simulink model "DDEF_Nylon_fwr"  (R2026a)
settings: Solver=ode45  StopTime=10  MaxStep=1e-4  RelTol=1e-6
undefined symbols (not defined in the file): RL
libraries: fl_lib x5, ee_lib x4, nesl_utility x4, simulink x1
settings Model: Creator=Satyanarayan  LastModifiedBy=Satyanarayan

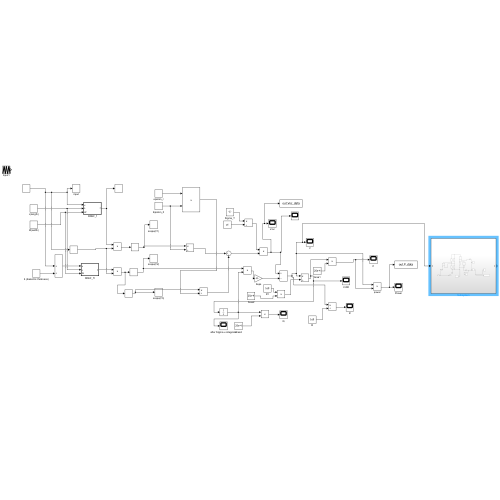
[thumbnail: Simulink's stored preview of the top-level diagram]
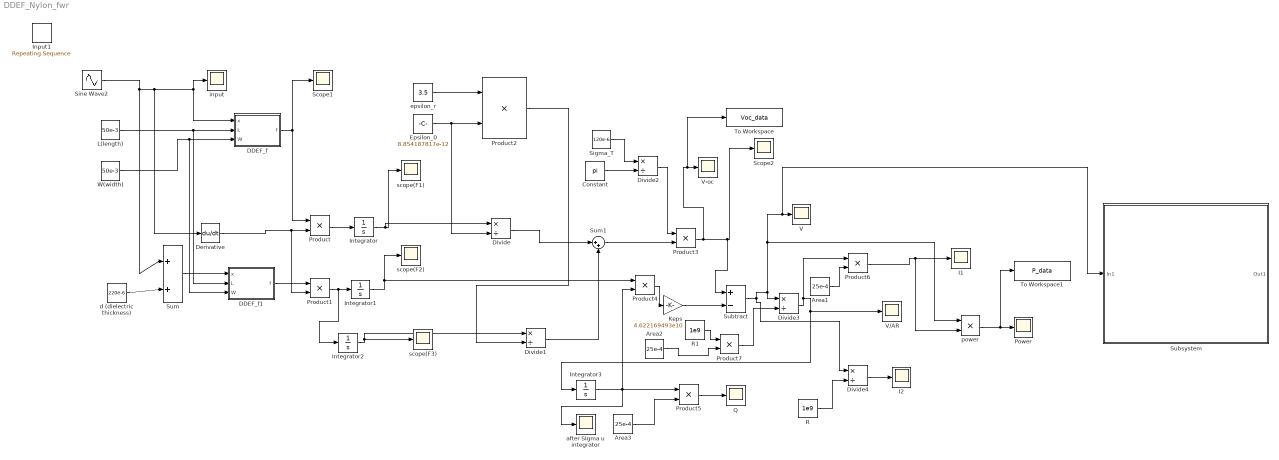
== system DDEF_Nylon_fwr ==
  Area1 : Constant  Value=25e-4
  Area2 : Constant  Value=25e-4
  Area3 : Constant  Value=25e-4
  Constant : Constant  Value=pi
  DDEF_f : MATLAB Function  TreatAsAtomicUnit=on
  DDEF_f1 : MATLAB Function  TreatAsAtomicUnit=on
  Derivative : Derivative
  Divide{,1..4} (5 alike) : Product  Inputs=*/
  Epsilon_0 : Constant  Value=8.854187817e-12
  I1 : Scope
      settings: ActiveDisplayYMinimum=-1  ActiveDisplayYMaximum=1  DataLoggingVariableName=ScopeData11
  I2 : Scope
      settings: ActiveDisplayYMinimum=-1  ActiveDisplayYMaximum=1  DataLoggingVariableName=ScopeData12
  Input1 : simulink/Sources/Repeating Sequence  rep_seq_t=[0 0.5 1]  rep_seq_y=[0 0.01 0]
  Integrator : Integrator
  Integrator1 : Integrator  InitialCondition=3.44206e-4
  Integrator2 : Integrator
  Integrator3 : Integrator
  Keps : Gain  Gain=4.622169493e10
  L(length) : Constant  Value=50e-3
  Power : Scope
      settings: ActiveDisplayYMinimum=-0.00046209975030593484  ActiveDisplayYMaximum=0.0041588977527534142  DataLoggingVariableName=ScopeData13
  Product{,1..7} (8 alike) : Product
  Q : Scope
      settings: ActiveDisplayYMinimum=-1  ActiveDisplayYMaximum=1  DataLoggingVariableName=ScopeData10
  R : Constant  Value=1e9
  R1 : Constant  Value=1e9
  Scope1 : Scope
      settings: ActiveDisplayYMinimum=0.392699081716402  ActiveDisplayYMaximum=1.7016960205353724
  Scope2 : Scope
      settings: ActiveDisplayYMinimum=-1  ActiveDisplayYMaximum=1  DataLoggingVariableName=ScopeData5
  Sigma_T : Constant  Value=120e-6
  Sine Wave2 : Sin  Amplitude=2.5e-3  Bias=2.5e-3  Frequency=2*pi  Phase=3*pi/2  SampleTime=0
  Subsystem : Subsystem
  Subtract : Sum  Inputs=+-
  Sum : Sum  Inputs=|++
  Sum1 : Sum  Inputs=|++
  To Workspace : ToWorkspace  VariableName=Voc_data  SaveFormat=Timeseries  SampleTime=-1
  To Workspace1 : ToWorkspace  VariableName=P_data  SaveFormat=Timeseries  SampleTime=-1
  V : Scope
      settings: ActiveDisplayYMinimum=-1408.9203660031535  ActiveDisplayYMaximum=2630.0910844886675  DataLoggingVariableName=ScopeData6
  V-oc : Scope
      settings: ActiveDisplayYMinimum=-4819.8788285773553  ActiveDisplayYMaximum=43269.459838287345  DataLoggingVariableName=ScopeData9
  V/AR : Scope
      settings: ActiveDisplayYMinimum=-1  ActiveDisplayYMaximum=1  DataLoggingVariableName=ScopeData8
  W(width) : Constant  Value=50e-3
  after SIgma u integrator : Scope
      settings: ActiveDisplayYMinimum=-3.4716855225550229E-6  ActiveDisplayYMaximum=3.1245169702995217E-5  DataLoggingVariableName=ScopeData7
  d (dielectric thickness) : Constant  Value=220e-6
  epsilon_r : Constant  Value=3.5
  input : Scope
      settings: ActiveDisplayYMinimum=-0.0012499995532938208  ActiveDisplayYMaximum=0.011249995979644389
  power : Product
  scope(F1) : Scope
      settings: ActiveDisplayYMinimum=-0.00121173424121706  ActiveDisplayYMaximum=0.01090560817095354  DataLoggingVariableName=ScopeData2
  scope(F2) : Scope
      settings: ActiveDisplayYMinimum=0.00041232627300281824  ActiveDisplayYMaximum=0.01127511879777789  DataLoggingVariableName=ScopeData3
  scope(F3) : Scope
      settings: ActiveDisplayYMinimum=-0.0010878737269972396  ActiveDisplayYMaximum=0.009774918797777957  DataLoggingVariableName=ScopeData4
  wires:
  Area1/1 -> Product6/2
  Divide2/1 -> Product3/1
  Product4/1 -> Keps/1
  Divide4/1 -> I2/1
  Divide/1 -> Sum1/1
  Sigma_T/1 -> Divide2/1
  Keps/1 -> Subtract/2
  Divide3/1 -> Product6/1, Integrator3/1, V/AR/1
  Sum/1 -> DDEF_f1/1(x)
  d (dielectric thickness)/1 -> Sum/2
  Product/1 -> Integrator/1
  Derivative/1 -> Product1/2, Product/2
  Integrator/1 -> Divide/1, scope(F1)/1
  Product3/1 -> To Workspace/1, V-oc/1, Subtract/1, Scope2/1
  Constant/1 -> Divide2/2
  Product7/1 -> Divide3/2
  Integrator2/1 -> Divide1/1, scope(F3)/1
  Product5/1 -> Q/1
  Sine Wave2/1 -> Sum/1, Derivative/1, DDEF_f/1(x), input/1
  R/1 -> Divide4/2
  power/1 -> To Workspace1/1, Power/1
  Area3/1 -> Product5/2
  Integrator3/1 -> Product5/1, after SIgma u integrator/1, Product4/2
  Subtract/1 -> Divide4/1, Subsystem/1(In1), V/1, power/1, Divide3/1
  Product1/1 -> Integrator2/1, Integrator1/1
  Product6/1 -> power/2, I1/1
  Product2/1 -> Divide1/2
  Divide1/1 -> Sum1/2
  L(length)/1 -> DDEF_f1/2(L), DDEF_f/2(L)
  Epsilon_0/1 -> Divide/2, Product2/2
  DDEF_f/1(f) -> Product/1, Scope1/1
  DDEF_f1/1(f) -> Product1/1
  Integrator1/1 -> Product4/1, scope(F2)/1
  Sum1/1 -> Product3/2
  W(width)/1 -> DDEF_f1/3(W), DDEF_f/3(W)
  epsilon_r/1 -> Product2/1
  R1/1 -> Product7/1
  Area2/1 -> Product7/2

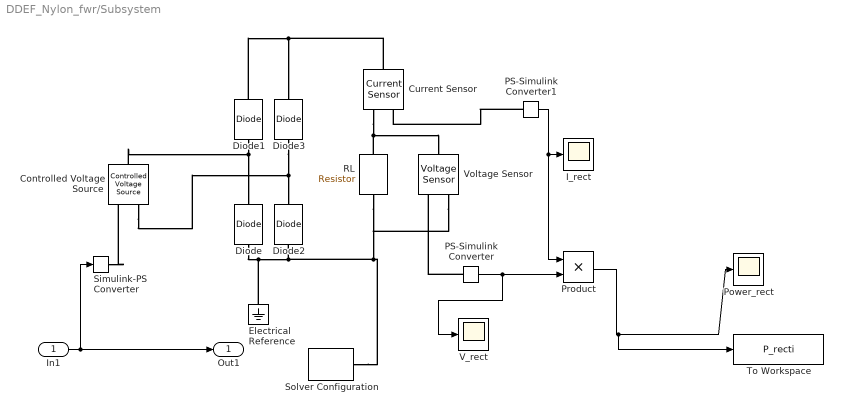
== system DDEF_Nylon_fwr/Subsystem ==
  In1 : Inport
  Controlled Voltage Source : fl_lib/Electrical/Electrical Sources/Controlled Voltage Source
  Current Sensor : fl_lib/Electrical/Electrical Sensors/Current Sensor
  Diode{,1..3} (4 alike) : ee_lib/Semiconductors & Converters/Diode  ModelType=ee.enum.diode.modelType.pwl  TableType=ee.enum.diode.tableType.IfMat  IfMat=[.07, .12, .19, 1.75, 4.24, 7.32, 11.2; .16, .3, .72, 2.14, 5.02, 8.35, 13.12] A  VfMat=[.9, 1.15, 1.25, 1.5, 1.75, 2.17, 2.6, 2.85; .58, .68, .75, 1.1, 1.38, 1.77, 2.27, 2.7] V  TjVec=[25, 125] degC  VfVec=[.5, .7, .9, 1.3, 1.7, 2.1, 2.5] V  IfVec=[.1, .2, .5, 1, 2, 4, 7, 10] A  IrMat=[1e-06, 2e-06, 5e-06, 1e-05, 2.5e-05, 5e-05, .0001; 2e-06, 5e-06, 1e-05, 4e-05, 8e-05, .0002, .0005] A  VrMat=[10, 100, 200, 250, 300, 325, 350; 10, 70, 160, 220, 270, 300, 320] V  VrVec=[10, 20, 40, 50, 70, 80, 100] V  IrVec=[1e-06, 2e-06, 5e-06, 1e-05, 2e-05, 5e-05, .0001] A  Vf=0.6 V  Ron=0.3 Ohm  Goff=1e-8 S  prmExp=ee.enum.diode.expParam.useTwo  I12=[.0137, .545] A  V12=[.6, .7] V  RS=0 Ohm  Tmeas=298.15 K  IS=1e-12 A  ec=1  I1=0.0137 A  V1=0.6 V  N_series=1  N_parallel=1  ZenerEnable=false  Rz=0.3 Ohm  BV=30 V  C_param=ee.enum.diode.capParam.fixed  CJ=0 pF  CJ0=5 pF  Vvec=[.1, 10, 100] V  Cvec=[3.5, 1, .4] pF  VJ=1 V  Mgrad=0.5  FC=0.5  Q_param=ee.enum.diode.recoveryParam.off  iRM=-7.15 A  iF=4 A  didt=-750 A/us  trr_factor=3  trr=115 ns  Qrr=150 nA*s  Vr=-600 V  Ls=150 nH  Erec=0.03 J  TT=50 ns  tau=100 ns  T_param=ee.enum.diode.temperatureParam.off  Tdevice=298.15 K  I1_T2=0.245 A  V1_T2=0.5 V  IS_T2=1.25e-7 A  Tmeas2=125 degC  XTI_param=ee.enum.diode.xtiParam.pn  XTI=3  EG_param=ee.enum.diode.egapParam.material_si  EG=1.11 eV  dBVdT=0 V/K  enable_fault_input=simscape.enum.onoff.off  i_specify=off  i_priority=None  i=0 A  i_nominal_specify=off  i_nominal_value=1  i_nominal_unit=A  v_specify=off  v_priority=None  v=0 V  v_nominal_specify=off  v_nominal_value=1  v_nominal_unit=V  v_capacitor_specify=off  v_capacitor_priority=None  v_capacitor=0 V  v_capacitor_nominal_specify=off  v_capacitor_nominal_value=1  v_capacitor_nominal_unit=V  Qj_specify=off  Qj_priority=High  Qj=0 C  Qj_nominal_specify=off  Qj_nominal_value=1  Qj_nominal_unit=C  i_diode_specify=off  i_diode_priority=None  i_diode=0 A  i_diode_nominal_specify=off  i_diode_nominal_value=1  i_diode_nominal_unit=A  v_diode_specify=off  v_diode_priority=None  v_diode=0 V  v_diode_nominal_specify=off  v_diode_nominal_value=1  v_diode_nominal_unit=V  i_capacitor_specify=off  i_capacitor_priority=None  i_capacitor=0 A  i_capacitor_nominal_specify=off  i_capacitor_nominal_value=1  i_capacitor_nominal_unit=A  fidelity_level=ee.enum.diode.fidelity.includeChargeDyn  rec_loss_model=ee.enum.diode.reverseRecoveryModelTabulateUpTo3D.fixed  ErecVal=0 J  scaleWithIandV=true  ErecMat=zeros(2, 3) J  ErecMat3D=zeros(2, 3, 2) J  TjrecVec=[298.15, 398.15] K  IfrecVec=[.1, 1, 10] A  IrecVal=10 A  VrecVal=10 V  VrecVec=[0, 100] V  tFilter=1 / 1000 / 100 s  thermal_network_parameterization=ee.enum.thermalNetworkTopology.junctionCase  Rth=[0, 10] K/W  Rth_Cauer=[1, 3, 10] K/W  Rth_Foster=[.08, .14, .22, .16] K/W  thermal_mass_parameterization=ee.enum.thermalNetwork.timeconstant  thermal_mass=[0, 1] J/K  thermal_mass_Cauer=[.1, .3, 1] J/K  thermal_mass_Foster=[.001, .005, .05, .5] J/K  thermal_time_constant=[0, 10] s  thermal_time_constant_Cauer=[1, 3, 10] s  thermal_time_constant_Foster=[7e-05, .0007, .01, .08] s  thermal_mass_initial_temperatures=[25, 25] degC  thermal_mass_initial_temperatures_Cauer=[25, 25, 25] degC  junction_thermal_mass=0.01 J/K  Tvec_initial_Foster=[25, 25, 25, 25] degC  no_thermal_network=0  junction_temperature_specify=off  junction_temperature_priority=None  junction_temperature=25 degC  junction_temperature_nominal_specify=off  junction_temperature_nominal_value=1  junction_temperature_nominal_unit=degC
  Electrical Reference : fl_lib/Electrical/Electrical Elements/Electrical Reference
  I_rect : Scope
      settings: ActiveDisplayYMinimum=-1  ActiveDisplayYMaximum=1  DataLoggingVariableName=ScopeData15
  PS-Simulink Converter : nesl_utility/PS-Simulink Converter  PhysicalDomain=network_engine_domain  SubClassName=ps_output  LeftPortType=input  RightPortType=output  PseudoPeriodic=off  Frequencies=[]  VectorFormat=inherit  Unit=inherit  AffineConversion=off
  PS-Simulink Converter1 : nesl_utility/PS-Simulink Converter  PhysicalDomain=network_engine_domain  SubClassName=ps_output  LeftPortType=input  RightPortType=output  PseudoPeriodic=off  Frequencies=[]  VectorFormat=inherit  Unit=inherit  AffineConversion=off
  Power_rect : Scope
      settings: ActiveDisplayYMinimum=-0.00061882252065740835  ActiveDisplayYMaximum=0.0055694026859166761  DataLoggingVariableName=ScopeData16
  Product : Product
  RL : fl_lib/Electrical/Electrical Elements/Resistor  R=RL Ohm  i_specify=off  i_priority=None  i=0 A  i_nominal_specify=off  i_nominal_value=1  i_nominal_unit=A  v_specify=off  v_priority=None  v=0 V  v_nominal_specify=off  v_nominal_value=1  v_nominal_unit=V
  Simulink-PS Converter : nesl_utility/Simulink-PS Converter  PhysicalDomain=network_engine_domain  SubClassName=ps_input  LeftPortType=input  RightPortType=output  PseudoPeriodic=off  Frequencies=[]  NoiseDistribution=none  NoiseParameters=[]  Unit=V  AffineConversion=off  FilteringAndDerivatives=provide  SimscapeFilterOrder=1  InputFilterTimeConstant=0.001  UdotUserProvided=0
  Solver Configuration : nesl_utility/Solver Configuration  PhysicalDomain=network_engine_domain  SubClassName=solver  LeftPortType=input  RightPortType=generic  Tones=[]  Harmonics=[]  SimulateNoise=off  Profile=off  UseLocalSampling=off  EnableSwitchedLinearOptims=on  FrequencyDomain=off  UseCCode=off  RelTol=0.001  AbsTol=0.001  MinStep=1e-09  ToWorkspace=off  RevertToSquareIcSolve=off  NumHomotopyIterations=100  PhasorMode=off  PhasorModeNumHarmonics=1  ConsistencySolver=NEWTON_XTOL_AFTER_FTOL  CanonicalOrdering=CANONICAL  OptimizeIntermediates=OPTIMIZED  IndexReductionMethod=DerivativeReplacement  DoDC=off  ResidualTolerance=1e-09  ConsistencyTolSource=GLOBAL  ConsistencyAbsTol=0.001  ConsistencyRelTol=0.001  ConsistencyTolFactor=0.001  UseLocalSolver=off  LocalSolverChoice=NE_BACKWARD_EULER_ADVANCER  ResolveIndetEquations=on  FunctionEvalNumThread=1  LocalSolverSampleTime=0.001  DoFixedCost=off  MaxNonlinIter=3  MaxModeIter=2  ComputeImpulses=off  ImpulseIterations=2  LinearAlgebra=auto  LinearAlgebraNumThread=0  EquationFormulation=NE_TIME_EF  DelaysMemoryBudget=1024  AutomaticFiltering=on  FilteringTimeConstant=0.001  PartitionStorageMethod=AS_NEEDED  PartitionMemoryBudget=1024  PartitionMethod=ROBUST  MultibodyUseLocalSolver=off  MultibodyLocalSolverChoice=ODE1  MultibodyLocalSolverSampleTime=0.001
  To Workspace : ToWorkspace  VariableName=P_recti  SaveFormat=Timeseries  SampleTime=-1
  V_rect : Scope
      settings: ActiveDisplayYMinimum=-278.14548549558316  ActiveDisplayYMaximum=2503.1160814490117  DataLoggingVariableName=ScopeData14
  Voltage Sensor : fl_lib/Electrical/Electrical Sensors/Voltage Sensor
  Out1 : Outport
  wires:
  In1/1 -> Simulink-PS Converter/1, Out1/1
  PS-Simulink Converter/1 -> V_rect/1, Product/2
  PS-Simulink Converter1/1 -> Product/1, I_rect/1
  Product/1 -> To Workspace/1, Power_rect/1
  connections:
  Diode1/RConn1 -- Diode3/RConn1 -- Current Sensor/LConn1
  Diode1/LConn1 -- Controlled Voltage Source/LConn1 -- Diode/RConn1
  Diode3/LConn1 -- Controlled Voltage Source/RConn2 -- Diode2/RConn1
  Diode/LConn1 -- Solver Configuration/RConn1 -- RL/RConn1 -- Voltage Sensor/RConn2 -- Diode2/LConn1 -- Electrical Reference/LConn1
  Simulink-PS Converter/RConn1 -- Controlled Voltage Source/RConn1
  PS-Simulink Converter/LConn1 -- Voltage Sensor/RConn1
  PS-Simulink Converter1/LConn1 -- Current Sensor/RConn1
  RL/LConn1 -- Current Sensor/RConn2 -- Voltage Sensor/LConn1

== matlab function DDEF_Nylon_fwr/DDEF_f ==
  data: x input; f output; L input; W input
function f = DDEF_f(x,L,W)

z = max(x,1e-12);

f = atan((L*W)/(2*z*sqrt(L^2 + W^2 + 4*z^2)));

end

== matlab function DDEF_Nylon_fwr/DDEF_f1 ==
  data: x input; f output; L input; W input
function f = DDEF_f(x,L,W)

z = max(x,1e-12);

f = atan((L*W)/(2*z*sqrt(L^2 + W^2 + 4*z^2)));

end
